simulink model "Sim"  (R2016a)
settings: Solver=VariableStepAuto  StartTime=0.0  StopTime=1500  FixedStep=1  RelTol=1e-3
values from neighbouring files (symbols this model uses):
  A = 7.841E16    (= 7.841e+16)    [Parameters.m]
  cv = 1820000    [Parameters.m]
  detaX = 0.0013333    [Parameters.m]
  Ea = 1.4766E5    (= 147660)    [Parameters.m]
  H_dr = 4.92E8    (= 492000000)    [Parameters.m]
  H_pc = 1.992E8    (= 199200000)    [Parameters.m]
  ord = 0.75    [Parameters.m]
  q_dot = 3.981E4    (= 39810)    [Parameters.m]
  T_0 = 298.15    [Parameters.m]
  Tl = 334.15    [Parameters.m]
  Ts = 331.15    [Parameters.m]
(part 3 of 3)

== system Sim/Heat treansfer13 ==
  Temp(+) : Inport
  Temp(-) : Inport  Port=2
  Gain14 : Gain  Gain=lamda/detaX/detaX
  Subtract : Sum  Inputs=+-
  Q[W/m3] : Outport
  wires:
  Temp(-)/1 -> Subtract/2
  Temp(+)/1 -> Subtract/1
  Subtract/1 -> Gain14/1  "Temp difference"
  Gain14/1 -> Q[W/m3]/1

== system Sim/Heat treansfer14 ==
  Temp(+) : Inport
  Temp(-) : Inport  Port=2
  Gain14 : Gain  Gain=lamda/detaX/detaX
  Subtract : Sum  Inputs=+-
  Q[W/m3] : Outport
  wires:
  Temp(-)/1 -> Subtract/2
  Temp(+)/1 -> Subtract/1
  Subtract/1 -> Gain14/1  "Temp difference"
  Gain14/1 -> Q[W/m3]/1

== system Sim/Heat treansfer15 ==
  Temp(+) : Inport
  Temp(-) : Inport  Port=2
  Gain14 : Gain  Gain=lamda/detaX/detaX
  Subtract : Sum  Inputs=+-
  Q[W/m3] : Outport
  wires:
  Temp(-)/1 -> Subtract/2
  Temp(+)/1 -> Subtract/1
  Subtract/1 -> Gain14/1  "Temp difference"
  Gain14/1 -> Q[W/m3]/1

== system Sim/Heat treansfer16 ==
  Temp(+) : Inport
  Temp(-) : Inport  Port=2
  Gain14 : Gain  Gain=lamda/detaX/detaX
  Subtract : Sum  Inputs=+-
  Q[W/m3] : Outport
  wires:
  Temp(-)/1 -> Subtract/2
  Temp(+)/1 -> Subtract/1
  Subtract/1 -> Gain14/1  "Temp difference"
  Gain14/1 -> Q[W/m3]/1

== system Sim/Heat treansfer17 ==
  Temp(+) : Inport
  Temp(-) : Inport  Port=2
  Gain14 : Gain  Gain=lamda/detaX/detaX
  Subtract : Sum  Inputs=+-
  Q[W/m3] : Outport
  wires:
  Temp(-)/1 -> Subtract/2
  Temp(+)/1 -> Subtract/1
  Subtract/1 -> Gain14/1  "Temp difference"
  Gain14/1 -> Q[W/m3]/1

== system Sim/Heat treansfer18 ==
  Temp(+) : Inport
  Temp(-) : Inport  Port=2
  Gain14 : Gain  Gain=lamda/detaX/detaX
  Subtract : Sum  Inputs=+-
  Q[W/m3] : Outport
  wires:
  Temp(-)/1 -> Subtract/2
  Temp(+)/1 -> Subtract/1
  Subtract/1 -> Gain14/1  "Temp difference"
  Gain14/1 -> Q[W/m3]/1

== system Sim/Heat treansfer19 ==
  Temp(+) : Inport
  Temp(-) : Inport  Port=2
  Gain14 : Gain  Gain=lamda/detaX/detaX
  Subtract : Sum  Inputs=+-
  Q[W/m3] : Outport
  wires:
  Temp(-)/1 -> Subtract/2
  Temp(+)/1 -> Subtract/1
  Subtract/1 -> Gain14/1  "Temp difference"
  Gain14/1 -> Q[W/m3]/1

== system Sim/Heat treansfer2 ==
  Temp(+) : Inport
  Temp(-) : Inport  Port=2
  Gain14 : Gain  Gain=lamda/detaX/detaX
  Subtract : Sum  Inputs=+-
  Q[W/m3] : Outport
  wires:
  Temp(-)/1 -> Subtract/2
  Temp(+)/1 -> Subtract/1
  Subtract/1 -> Gain14/1  "Temp difference"
  Gain14/1 -> Q[W/m3]/1

== system Sim/Heat treansfer20 ==
  Temp(+) : Inport
  Temp(-) : Inport  Port=2
  Gain14 : Gain  Gain=lamda/detaX/detaX
  Subtract : Sum  Inputs=+-
  Q[W/m3] : Outport
  wires:
  Temp(-)/1 -> Subtract/2
  Temp(+)/1 -> Subtract/1
  Subtract/1 -> Gain14/1  "Temp difference"
  Gain14/1 -> Q[W/m3]/1

== system Sim/Heat treansfer21 ==
  Temp(+) : Inport
  Temp(-) : Inport  Port=2
  Gain14 : Gain  Gain=lamda/detaX/detaX
  Subtract : Sum  Inputs=+-
  Q[W/m3] : Outport
  wires:
  Temp(-)/1 -> Subtract/2
  Temp(+)/1 -> Subtract/1
  Subtract/1 -> Gain14/1  "Temp difference"
  Gain14/1 -> Q[W/m3]/1

== system Sim/Heat treansfer22 ==
  Temp(+) : Inport
  Temp(-) : Inport  Port=2
  Gain14 : Gain  Gain=lamda/detaX/detaX
  Subtract : Sum  Inputs=+-
  Q[W/m3] : Outport
  wires:
  Temp(-)/1 -> Subtract/2
  Temp(+)/1 -> Subtract/1
  Subtract/1 -> Gain14/1  "Temp difference"
  Gain14/1 -> Q[W/m3]/1

== system Sim/Heat treansfer23 ==
  Temp(+) : Inport
  Temp(-) : Inport  Port=2
  Gain14 : Gain  Gain=lamda/detaX/detaX
  Subtract : Sum  Inputs=+-
  Q[W/m3] : Outport
  wires:
  Temp(-)/1 -> Subtract/2
  Temp(+)/1 -> Subtract/1
  Subtract/1 -> Gain14/1  "Temp difference"
  Gain14/1 -> Q[W/m3]/1

== system Sim/Heat treansfer24 ==
  Temp(+) : Inport
  Temp(-) : Inport  Port=2
  Gain14 : Gain  Gain=lamda/detaX/detaX
  Subtract : Sum  Inputs=+-
  Q[W/m3] : Outport
  wires:
  Temp(-)/1 -> Subtract/2
  Temp(+)/1 -> Subtract/1
  Subtract/1 -> Gain14/1  "Temp difference"
  Gain14/1 -> Q[W/m3]/1

== system Sim/Heat treansfer25 ==
  Temp(+) : Inport
  Temp(-) : Inport  Port=2
  Gain14 : Gain  Gain=lamda/detaX/detaX
  Subtract : Sum  Inputs=+-
  Q[W/m3] : Outport
  wires:
  Temp(-)/1 -> Subtract/2
  Temp(+)/1 -> Subtract/1
  Subtract/1 -> Gain14/1  "Temp difference"
  Gain14/1 -> Q[W/m3]/1

== system Sim/Heat treansfer26 ==
  Temp(+) : Inport
  Temp(-) : Inport  Port=2
  Gain14 : Gain  Gain=lamda/detaX/detaX
  Subtract : Sum  Inputs=+-
  Q[W/m3] : Outport
  wires:
  Temp(-)/1 -> Subtract/2
  Temp(+)/1 -> Subtract/1
  Subtract/1 -> Gain14/1  "Temp difference"
  Gain14/1 -> Q[W/m3]/1

== system Sim/Heat treansfer27 ==
  Temp(+) : Inport
  Temp(-) : Inport  Port=2
  Gain14 : Gain  Gain=lamda/detaX/detaX
  Subtract : Sum  Inputs=+-
  Q[W/m3] : Outport
  wires:
  Temp(-)/1 -> Subtract/2
  Temp(+)/1 -> Subtract/1
  Subtract/1 -> Gain14/1  "Temp difference"
  Gain14/1 -> Q[W/m3]/1

== system Sim/Heat treansfer28 ==
  Temp(+) : Inport
  Temp(-) : Inport  Port=2
  Gain14 : Gain  Gain=lamda/detaX/detaX
  Subtract : Sum  Inputs=+-
  Q[W/m3] : Outport
  wires:
  Temp(-)/1 -> Subtract/2
  Temp(+)/1 -> Subtract/1
  Subtract/1 -> Gain14/1  "Temp difference"
  Gain14/1 -> Q[W/m3]/1

== system Sim/Heat treansfer29 ==
  Temp(+) : Inport
  Temp(-) : Inport  Port=2
  Gain14 : Gain  Gain=lamda/detaX/detaX
  Subtract : Sum  Inputs=+-
  Q[W/m3] : Outport
  wires:
  Temp(-)/1 -> Subtract/2
  Temp(+)/1 -> Subtract/1
  Subtract/1 -> Gain14/1  "Temp difference"
  Gain14/1 -> Q[W/m3]/1

== system Sim/Heat treansfer3 ==
  Temp(+) : Inport
  Temp(-) : Inport  Port=2
  Gain14 : Gain  Gain=lamda/detaX/detaX
  Subtract : Sum  Inputs=+-
  Q[W/m3] : Outport
  wires:
  Temp(-)/1 -> Subtract/2
  Temp(+)/1 -> Subtract/1
  Subtract/1 -> Gain14/1  "Temp difference"
  Gain14/1 -> Q[W/m3]/1

== system Sim/Heat treansfer30 ==
  Temp(+) : Inport
  Temp(-) : Inport  Port=2
  Gain14 : Gain  Gain=lamda/detaX/detaX
  Subtract : Sum  Inputs=+-
  Q[W/m3] : Outport
  wires:
  Temp(-)/1 -> Subtract/2
  Temp(+)/1 -> Subtract/1
  Subtract/1 -> Gain14/1  "Temp difference"
  Gain14/1 -> Q[W/m3]/1

== system Sim/Heat treansfer31 ==
  Temp(+) : Inport
  Temp(-) : Inport  Port=2
  Gain14 : Gain  Gain=lamda/detaX/detaX
  Subtract : Sum  Inputs=+-
  Q[W/m3] : Outport
  wires:
  Temp(-)/1 -> Subtract/2
  Temp(+)/1 -> Subtract/1
  Subtract/1 -> Gain14/1  "Temp difference"
  Gain14/1 -> Q[W/m3]/1

== system Sim/Heat treansfer32 ==
  Temp(+) : Inport
  Temp(-) : Inport  Port=2
  Gain14 : Gain  Gain=lamda/detaX/detaX
  Subtract : Sum  Inputs=+-
  Q[W/m3] : Outport
  wires:
  Temp(-)/1 -> Subtract/2
  Temp(+)/1 -> Subtract/1
  Subtract/1 -> Gain14/1  "Temp difference"
  Gain14/1 -> Q[W/m3]/1

== system Sim/Heat treansfer33 ==
  Temp(+) : Inport
  Temp(-) : Inport  Port=2
  Gain14 : Gain  Gain=lamda/detaX/detaX
  Subtract : Sum  Inputs=+-
  Q[W/m3] : Outport
  wires:
  Temp(-)/1 -> Subtract/2
  Temp(+)/1 -> Subtract/1
  Subtract/1 -> Gain14/1  "Temp difference"
  Gain14/1 -> Q[W/m3]/1

== system Sim/Heat treansfer34 ==
  Temp(+) : Inport
  Temp(-) : Inport  Port=2
  Gain14 : Gain  Gain=lamda/detaX/detaX
  Subtract : Sum  Inputs=+-
  Q[W/m3] : Outport
  wires:
  Temp(-)/1 -> Subtract/2
  Temp(+)/1 -> Subtract/1
  Subtract/1 -> Gain14/1  "Temp difference"
  Gain14/1 -> Q[W/m3]/1

== system Sim/Heat treansfer35 ==
  Temp(+) : Inport
  Temp(-) : Inport  Port=2
  Gain14 : Gain  Gain=lamda/detaX/detaX
  Subtract : Sum  Inputs=+-
  Q[W/m3] : Outport
  wires:
  Temp(-)/1 -> Subtract/2
  Temp(+)/1 -> Subtract/1
  Subtract/1 -> Gain14/1  "Temp difference"
  Gain14/1 -> Q[W/m3]/1

== system Sim/Heat treansfer36 ==
  Temp(+) : Inport
  Temp(-) : Inport  Port=2
  Gain14 : Gain  Gain=lamda/detaX/detaX
  Subtract : Sum  Inputs=+-
  Q[W/m3] : Outport
  wires:
  Temp(-)/1 -> Subtract/2
  Temp(+)/1 -> Subtract/1
  Subtract/1 -> Gain14/1  "Temp difference"
  Gain14/1 -> Q[W/m3]/1

== system Sim/Heat treansfer37 ==
  Temp(+) : Inport
  Temp(-) : Inport  Port=2
  Gain14 : Gain  Gain=lamda/detaX/detaX
  Subtract : Sum  Inputs=+-
  Q[W/m3] : Outport
  wires:
  Temp(-)/1 -> Subtract/2
  Temp(+)/1 -> Subtract/1
  Subtract/1 -> Gain14/1  "Temp difference"
  Gain14/1 -> Q[W/m3]/1

== system Sim/Heat treansfer38 ==
  Temp(+) : Inport
  Temp(-) : Inport  Port=2
  Gain14 : Gain  Gain=lamda/detaX/detaX
  Subtract : Sum  Inputs=+-
  Q[W/m3] : Outport
  wires:
  Temp(-)/1 -> Subtract/2
  Temp(+)/1 -> Subtract/1
  Subtract/1 -> Gain14/1  "Temp difference"
  Gain14/1 -> Q[W/m3]/1

== system Sim/Heat treansfer39 ==
  Temp(+) : Inport
  Temp(-) : Inport  Port=2
  Gain14 : Gain  Gain=lamda/detaX/detaX
  Subtract : Sum  Inputs=+-
  Q[W/m3] : Outport
  wires:
  Temp(-)/1 -> Subtract/2
  Temp(+)/1 -> Subtract/1
  Subtract/1 -> Gain14/1  "Temp difference"
  Gain14/1 -> Q[W/m3]/1

== system Sim/Heat treansfer4 ==
  Temp(+) : Inport
  Temp(-) : Inport  Port=2
  Gain14 : Gain  Gain=lamda/detaX/detaX
  Subtract : Sum  Inputs=+-
  Q[W/m3] : Outport
  wires:
  Temp(-)/1 -> Subtract/2
  Temp(+)/1 -> Subtract/1
  Subtract/1 -> Gain14/1  "Temp difference"
  Gain14/1 -> Q[W/m3]/1

== system Sim/Heat treansfer40 ==
  Temp(+) : Inport
  Temp(-) : Inport  Port=2
  Gain14 : Gain  Gain=lamda/detaX/detaX
  Subtract : Sum  Inputs=+-
  Q[W/m3] : Outport
  wires:
  Temp(-)/1 -> Subtract/2
  Temp(+)/1 -> Subtract/1
  Subtract/1 -> Gain14/1  "Temp difference"
  Gain14/1 -> Q[W/m3]/1

== system Sim/Heat treansfer41 ==
  Temp(+) : Inport
  Temp(-) : Inport  Port=2
  Gain14 : Gain  Gain=lamda/detaX/detaX
  Subtract : Sum  Inputs=+-
  Q[W/m3] : Outport
  wires:
  Temp(-)/1 -> Subtract/2
  Temp(+)/1 -> Subtract/1
  Subtract/1 -> Gain14/1  "Temp difference"
  Gain14/1 -> Q[W/m3]/1

== system Sim/Heat treansfer42 ==
  Temp(+) : Inport
  Temp(-) : Inport  Port=2
  Gain14 : Gain  Gain=lamda/detaX/detaX
  Subtract : Sum  Inputs=+-
  Q[W/m3] : Outport
  wires:
  Temp(-)/1 -> Subtract/2
  Temp(+)/1 -> Subtract/1
  Subtract/1 -> Gain14/1  "Temp difference"
  Gain14/1 -> Q[W/m3]/1

== system Sim/Heat treansfer44 ==
  Temp(+) : Inport
  Temp(-) : Inport  Port=2
  Gain14 : Gain  Gain=lamda/detaX/detaX
  Subtract : Sum  Inputs=+-
  Q[W/m3] : Outport
  wires:
  Temp(-)/1 -> Subtract/2
  Temp(+)/1 -> Subtract/1
  Subtract/1 -> Gain14/1  "Temp difference"
  Gain14/1 -> Q[W/m3]/1

== system Sim/Heat treansfer5 ==
  Temp(+) : Inport
  Temp(-) : Inport  Port=2
  Gain14 : Gain  Gain=lamda/detaX/detaX
  Subtract : Sum  Inputs=+-
  Q[W/m3] : Outport
  wires:
  Temp(-)/1 -> Subtract/2
  Temp(+)/1 -> Subtract/1
  Subtract/1 -> Gain14/1  "Temp difference"
  Gain14/1 -> Q[W/m3]/1

== system Sim/Heat treansfer6 ==
  Temp(+) : Inport
  Temp(-) : Inport  Port=2
  Gain14 : Gain  Gain=lamda/detaX/detaX
  Subtract : Sum  Inputs=+-
  Q[W/m3] : Outport
  wires:
  Temp(-)/1 -> Subtract/2
  Temp(+)/1 -> Subtract/1
  Subtract/1 -> Gain14/1  "Temp difference"
  Gain14/1 -> Q[W/m3]/1

== system Sim/Heat treansfer7 ==
  Temp(+) : Inport
  Temp(-) : Inport  Port=2
  Gain14 : Gain  Gain=lamda/detaX/detaX
  Subtract : Sum  Inputs=+-
  Q[W/m3] : Outport
  wires:
  Temp(-)/1 -> Subtract/2
  Temp(+)/1 -> Subtract/1
  Subtract/1 -> Gain14/1  "Temp difference"
  Gain14/1 -> Q[W/m3]/1

== system Sim/Heat treansfer8 ==
  Temp(+) : Inport
  Temp(-) : Inport  Port=2
  Gain14 : Gain  Gain=lamda/detaX/detaX
  Subtract : Sum  Inputs=+-
  Q[W/m3] : Outport
  wires:
  Temp(-)/1 -> Subtract/2
  Temp(+)/1 -> Subtract/1
  Subtract/1 -> Gain14/1  "Temp difference"
  Gain14/1 -> Q[W/m3]/1

== system Sim/Heat treansfer9 ==
  Temp(+) : Inport
  Temp(-) : Inport  Port=2
  Gain14 : Gain  Gain=lamda/detaX/detaX
  Subtract : Sum  Inputs=+-
  Q[W/m3] : Outport
  wires:
  Temp(-)/1 -> Subtract/2
  Temp(+)/1 -> Subtract/1
  Subtract/1 -> Gain14/1  "Temp difference"
  Gain14/1 -> Q[W/m3]/1
